simulink model "UDP1"  (R2013b)
settings: Solver=ode45  StartTime=0.0  StopTime=100  MaxStep=0.01  MinStep=0.01  RelTol=1e-3
libraries: xpclib x2, dspnetwork x2, etargetslib x1
settings Model: Creator=lankuohsing  LastModifiedBy=lankuohsing
settings SolverCC: InitialStep=0.01

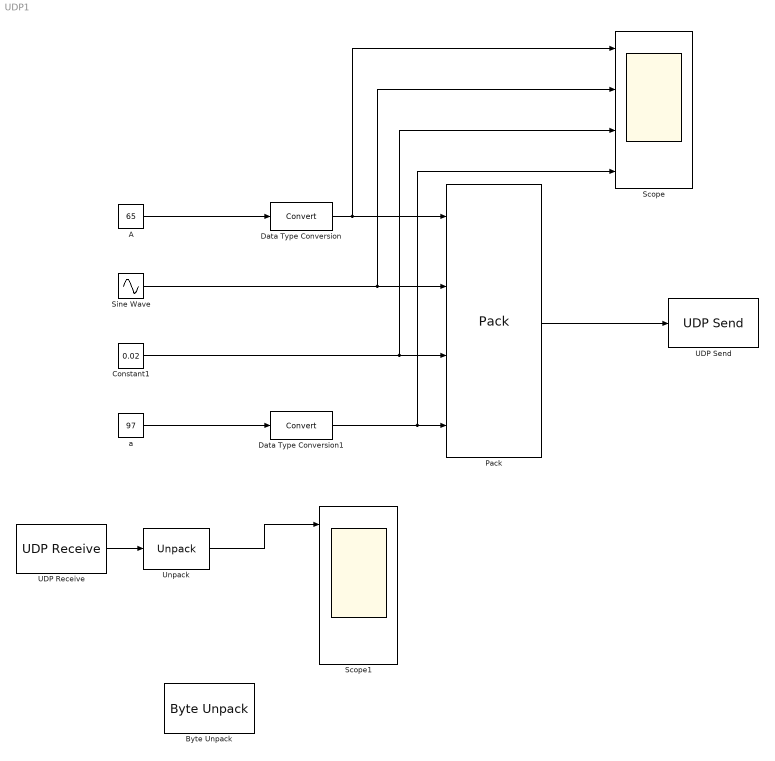
== system UDP1 ==
  A : Constant  Value=65
  Byte Unpack : etargetslib/Byte Unpack  dimensions={[1]}  datatypes={'double'}  byteAlign=1
  Constant1 : Constant  Value=0.02
  Data Type Conversion : DataTypeConversion
  Data Type Conversion1 : DataTypeConversion
  Pack : xpclib/UDP/Pack  datatypes={'uint8','double','double','uint8'}  byteAlign=1
  Scope : Scope  NumInputPorts=4
      settings: YMin=-5~-5~-5~-5  YMax=5~5~5~5
  Scope1 : Scope  NumInputPorts=4
      settings: YMin=-5~-5~-5~-5  YMax=5~5~5~5
  Sine Wave : Sin  SampleTime=0
  UDP Receive : dspnetwork/UDP Receive  localURL='0.0.0.0'  localPort=9090  remoteURL='127.0.0.1'  remotePort=-1  recvBufferSize=8192  dims=255  signalDatatype=uint8  isVarSize=on  showBlockingTime=on  blockingTime=inf  sampletime=0.01  blockPlatform=HOST
  UDP Send : dspnetwork/UDP Send  remoteURL='127.0.0.1'  remotePort=9090  localURL='0.0.0.0'  localPortSource=Automatically determine  localPort=-1  sampletime=-1  blockPlatform=HOST  separateLengthPort=0
  Unpack : xpclib/UDP/Unpack  dimensions={[1]}  datatypes={'uint8'}  byteAlign=1
  a : Constant  Value=97
  wires:
  A/1 -> Data Type Conversion/1
  Sine Wave/1 -> Pack/2, Scope/2
  Constant1/1 -> Scope/3, Pack/3
  Data Type Conversion1/1 -> Scope/4, Pack/4
  a/1 -> Data Type Conversion1/1
  Pack/1 -> UDP Send/1
  Data Type Conversion/1 -> Pack/1, Scope/1
  UDP Receive/1 -> Unpack/1
  Unpack/1 -> Scope1/1
